simulink model "P2_SIL_Model_Diag"  (R2016a)
settings: Solver=ode2  StartTime=0.0  StopTime=Cycle_End  RelTol=1e-3
undefined symbols (not defined in the file): air, APP1_OOR, APP2_OOR, APP_Conversion_IN, APP_Mismatch, bms_inletair_temp, bms_maxchargecurrent, bms_maxdischargecurrent, BMS_Notfallkuehlung, BPP_Flt, cal, clt, ClutchEngag, CrankRequest, dcdc, eng, Engine, EngOverTemp, ENGTRQ_MSMCH_Degraded_CP, ENGTRQ_MSMCH_ErrCritical_CP, ENGTRQ_MSMCH_LimpHome_CP, EngTrqMismatch, env, ess, ESS, ESSOverTemp, fd, FFD, g, gb, Grade, IMG, KeyPos_Flt, KeyPosition, lib_APP_Conversion_IN, lib_ESS_plant_V1_2, lib_OBC_Manager, LossCAN, max_vehicle_rad_air_flow, MCUOverTemp, mot, MotDirMismatch, MotOverTemp, MotTrqMismatch, mph2kph, mph2ms, NeutralGear, obc, OBC_Manager, ParkGear, PRNDL_Flt, ReverseGear, RFD, rho, ShiftLeverPosition, sigbuilder_block, Speed, t_amb, time, tloop ... (+2)
libraries: simulink x104, EC2_libraries x12, Diagnostic x11, lib_CANerror_Detect x3, Utility x1
(part 10 of 11)

== system P2_SIL_Model_Diag/Controller/HSC/Camaro Fault Detection/Input Conversions/MCU_Conversions/Override  rollingAliveCnt [123] ==
  note: Override Switch Subsystem
  note: This subsystem is used to override the model value of a signal to a constant value
  In1 : Inport
  Multiport Switch : MultiPortSwitch  DataPortOrder=Zero-based contiguous  Inputs=2  zeroidx=on
  Override Value : Constant  Value=0  OutDataTypeStr=double
  Signal Override Switch 0 = Use Model 1 = Use Constant : Constant  Value=0
  Out1 : Outport
  wires:
  Override Value/1 -> Multiport Switch/3
  Multiport Switch/1 -> Out1/1
  In1/1 -> Multiport Switch/2
  Signal Override Switch 0 = Use Model 1 = Use Constant/1 -> Multiport Switch/1

== system P2_SIL_Model_Diag/Controller/HSC/Camaro Fault Detection/Input Conversions/TCM_Conversions/Override  rollingAliveCnt [123] ==
  note: This subsystem is used to override the model value of a signal to a constant value
  note: Override Switch Subsystem
  In1 : Inport
  Multiport Switch : MultiPortSwitch  DataPortOrder=Zero-based contiguous  Inputs=2  zeroidx=on
  Override Value : Constant  Value=0  OutDataTypeStr=double
  Signal Override Switch 0 = Use Model 1 = Use Constant : Constant  Value=0
  Out1 : Outport
  wires:
  Signal Override Switch 0 = Use Model 1 = Use Constant/1 -> Multiport Switch/1
  In1/1 -> Multiport Switch/2
  Multiport Switch/1 -> Out1/1
  Override Value/1 -> Multiport Switch/3

== system P2_SIL_Model_Diag/Controller/HSC/Camaro Fault Detection/Input Conversions/TCM_Conversions/TCM_Rolling ==
  Constant8 : Constant
  Rolling Alive Counter1 : Stateflow chart  TreatAsAtomicUnit=on
  Switch1 : Switch  Criteria=u2 > Threshold
  Out1 : Outport
  wires:
  Switch1/1 -> Out1/1  "TCMRollingAliveCnt [0 1 2 3]"
  [TCM_CAN_fault] -> Switch1/2
  Rolling Alive Counter1/1(RollingAliveCnt) -> Switch1/3
  Constant8/1 -> Switch1/1

== system P2_SIL_Model_Diag/Controller/HSC/Camaro Fault Detection/Signal Diagnostic/Clutch Signal Diagnostic/Override  Engage ==
  note: This subsystem is used to override the model value of a signal to a constant value
  note: Override Switch Subsystem
  In1 : Inport
  Multiport Switch : MultiPortSwitch  DataPortOrder=Zero-based contiguous  Inputs=2  zeroidx=on
  Override Value : Constant  Value=0  OutDataTypeStr=double
  Signal Override Switch 0 = Use Model 1 = Use Constant : Constant
  Out1 : Outport
  wires:
  Signal Override Switch 0 = Use Model 1 = Use Constant/1 -> Multiport Switch/1
  In1/1 -> Multiport Switch/2
  Multiport Switch/1 -> Out1/1
  Override Value/1 -> Multiport Switch/3

== system P2_SIL_Model_Diag/Controller/HSC/Camaro Fault Detection/Signal Diagnostic/Clutch Signal Diagnostic/Rolling Alive Counter Detection ==
  In1 : Inport
  Chart : Stateflow chart  TreatAsAtomicUnit=on
  Constant : Constant  Value=0.01
  Detect Change : simulink/Logic and Bit Operations/Detect Change  vinit=1  InputProcessing=Inherited  OutDataTypeStr=boolean
  Out1 : Outport
  wires:
  In1/1 -> Detect Change/1
  Detect Change/1 -> Chart/1(PulseDetect)
  Chart/1(flag) -> Out1/1
  Constant/1 -> Chart/2(CycleTime)

== system P2_SIL_Model_Diag/Controller/HSC/Camaro Fault Detection/Signal Diagnostic/Driver Signal Diagnostic/APP_Crosscheck ==
  In1 : Inport
  In2 : Inport  Port=2
  Abs : Abs
  Compare To Constant : simulink/Logic and Bit Operations/Compare To Constant  relop=<=  const=0.1  OutDataTypeStr=boolean
  Sum : Sum  Inputs=+-
  Out1 : Outport
  wires:
  Sum/1 -> Abs/1
  Abs/1 -> Compare To Constant/1
  In1/1 -> Sum/1
  In2/1 -> Sum/2
  Compare To Constant/1 -> Out1/1  "Drv_APP_Agree"

== system P2_SIL_Model_Diag/Controller/HSC/Camaro Fault Detection/Signal Diagnostic/Driver Signal Diagnostic/Braking fail to decelerate ==
  In1 : Inport
  In2 : Inport  Port=2
  Compare To Constant : simulink/Logic and Bit Operations/Compare To Constant  relop=~=  const=50  OutDataTypeStr=boolean
  Constant2 : Constant  Value=0
  Gain : Gain  Gain=1/13
  Gain1 : Gain  Gain=10
  Relational Operator : RelationalOperator  Operator=>  OutDataTypeStr=boolean
  Switch : Switch  Threshold=1
  Out1 : Outport
  wires:
  Relational Operator/1 -> Out1/1
  In2/1 -> Switch/1
  In1/1 -> Compare To Constant/1
  Compare To Constant/1 -> Switch/2
  [chas_plant_lin_accel] -> Gain1/1
  Gain/1 -> Relational Operator/1
  Gain1/1 -> Relational Operator/2
  Switch/1 -> Gain/1  "0-20"
  Constant2/1 -> Switch/3

== system P2_SIL_Model_Diag/Controller/HSC/Camaro Fault Detection/Signal Diagnostic/Driver Signal Diagnostic/Latch ==
  In1 : Inport
  In2 : Inport  Port=2
  Memory : Memory
  NOT : Logic  Operator=NOT  OutDataTypeStr=boolean
  OR : Logic  OutDataTypeStr=boolean
  OR1 : Logic  Operator=OR  OutDataTypeStr=boolean
  Out1 : Outport
  wires:
  In1/1 -> OR1/1
  OR/1 -> OR1/2
  OR1/1 -> Out1/1, Memory/1
  NOT/1 -> OR/1
  Memory/1 -> OR/2
  In2/1 -> NOT/1

== system P2_SIL_Model_Diag/Controller/HSC/Camaro Fault Detection/Signal Diagnostic/ESS Signal Diagnostic/Rolling Alive Counter Detection ==
  In1 : Inport
  Chart : Stateflow chart  TreatAsAtomicUnit=on
  Constant : Constant  Value=0.01
  Constant1 : Constant  Value=0.01
  Detect Change : simulink/Logic and Bit Operations/Detect Change  vinit=1  InputProcessing=Inherited  OutDataTypeStr=boolean
  Out1 : Outport
  wires:
  Constant/1 -> Chart/2(CycleTime)
  Chart/1(flag) -> Out1/1
  Detect Change/1 -> Chart/1(PulseDetect)
  In1/1 -> Detect Change/1
  Constant1/1 -> Chart/3(tloop)

== system P2_SIL_Model_Diag/Controller/HSC/Camaro Fault Detection/Signal Diagnostic/ESS Signal Diagnostic/essSOCValidity_Check ==
  In1 : Inport
  Above Normal Operation : simulink/Logic and Bit Operations/Compare To Constant  relop===  const=3  OutDataTypeStr=boolean
  Below Normal Operation : simulink/Logic and Bit Operations/Compare To Constant  relop===  const=0  OutDataTypeStr=boolean
  Logical Operator : Logic  Operator=OR  AllPortsSameDT=off  OutDataTypeStr=boolean
  Logical Operator1 : Logic  Operator=NOT  AllPortsSameDT=off  OutDataTypeStr=boolean
  Out1 : Outport
  wires:
  Logical Operator1/1 -> Out1/1
  Above Normal Operation/1 -> Logical Operator/2
  Below Normal Operation/1 -> Logical Operator/1
  Logical Operator/1 -> Logical Operator1/1
  In1/1 -> Below Normal Operation/1, Above Normal Operation/1

== system P2_SIL_Model_Diag/Controller/HSC/Camaro Fault Detection/Signal Diagnostic/ESS Signal Diagnostic/essTsignalValidity_Check ==
  In1 : Inport
  Above Normal Operation : simulink/Logic and Bit Operations/Compare To Constant  relop===  const=4  OutDataTypeStr=boolean
  Below Normal Operation : simulink/Logic and Bit Operations/Compare To Constant  relop===  const=0  OutDataTypeStr=boolean
  Logical Operator : Logic  Operator=OR  AllPortsSameDT=off  OutDataTypeStr=boolean
  Logical Operator1 : Logic  Operator=NOT  AllPortsSameDT=off  OutDataTypeStr=boolean
  Out1 : Outport
  wires:
  In1/1 -> Above Normal Operation/1, Below Normal Operation/1
  Logical Operator/1 -> Logical Operator1/1
  Below Normal Operation/1 -> Logical Operator/1
  Above Normal Operation/1 -> Logical Operator/2
  Logical Operator1/1 -> Out1/1

== system P2_SIL_Model_Diag/Controller/HSC/Camaro Fault Detection/Signal Diagnostic/Engine Signal Diagnostic/EngTempValidity_Check ==
  In1 : Inport
  Above Normal Operation : simulink/Logic and Bit Operations/Compare To Constant  relop===  const=3  OutDataTypeStr=boolean
  Logical Operator1 : Logic  Operator=NOT  AllPortsSameDT=off  OutDataTypeStr=boolean
  Out1 : Outport
  wires:
  In1/1 -> Above Normal Operation/1
  Above Normal Operation/1 -> Logical Operator1/1
  Logical Operator1/1 -> Out1/1

== system P2_SIL_Model_Diag/Controller/HSC/Camaro Fault Detection/Signal Diagnostic/Engine Signal Diagnostic/Rolling Alive Counter Detection1 ==
  In1 : Inport
  Chart : Stateflow chart  TreatAsAtomicUnit=on
  Constant : Constant  Value=0.01
  Detect Change : simulink/Logic and Bit Operations/Detect Change  vinit=1  InputProcessing=Inherited  OutDataTypeStr=boolean
  Out1 : Outport
  wires:
  In1/1 -> Detect Change/1
  Detect Change/1 -> Chart/1(PulseDetect)
  Chart/1(flag) -> Out1/1
  Constant/1 -> Chart/2(CycleTime)

== system P2_SIL_Model_Diag/Controller/HSC/Camaro Fault Detection/Signal Diagnostic/Motor Signal Diagnostic/Rolling Alive Counter Detection ==
  In1 : Inport
  Chart : Stateflow chart  TreatAsAtomicUnit=on
  Constant : Constant  Value=0.01
  Detect Change : simulink/Logic and Bit Operations/Detect Change  vinit=1  InputProcessing=Inherited  OutDataTypeStr=boolean
  Out1 : Outport
  wires:
  Constant/1 -> Chart/2(CycleTime)
  Chart/1(flag) -> Out1/1
  Detect Change/1 -> Chart/1(PulseDetect)
  In1/1 -> Detect Change/1

== system P2_SIL_Model_Diag/Controller/HSC/Camaro Fault Detection/Signal Diagnostic/Motor Signal Diagnostic/Subsystem ==
  ClearFault : Inport
  In2 : Inport  Port=2
  MCUTempValidityCheck : simulink/Logic and Bit Operations/Interval Test  IntervalClosedRight=on  uplimit=100  IntervalClosedLeft=on  lowlimit=-40  OutDataTypeStr=boolean
  MCUTsignalRange : Stateflow chart  TreatAsAtomicUnit=on
  MCUTemp_degC_SigValid : Outport
  MCUTempRange : Outport  Port=2
  wires:
  In2/1 -> MCUTempValidityCheck/1, MCUTsignalRange/2(signalValue)
  ClearFault/1 -> MCUTsignalRange/1(clearFaults)
  MCUTempValidityCheck/1 -> MCUTemp_degC_SigValid/1  "MCUTemp_degC_SigValid"
  MCUTsignalRange/1(MCUTempRange) -> MCUTempRange/1  "MCUTempRange[0_4]"

== system P2_SIL_Model_Diag/Controller/HSC/Camaro Fault Detection/Signal Diagnostic/Motor Signal Diagnostic/Subsystem1 ==
  ClearFault : Inport
  In2 : Inport  Port=2
  MotorTempValidityCheck : simulink/Logic and Bit Operations/Interval Test  IntervalClosedRight=on  uplimit=150  IntervalClosedLeft=on  lowlimit=-20  OutDataTypeStr=boolean
  MotorTsignalRange : Stateflow chart  TreatAsAtomicUnit=on
  MotorTemp_degC_SigValid : Outport
  MotorTempRange : Outport  Port=2
  wires:
  ClearFault/1 -> MotorTsignalRange/1(clearFaults)
  MotorTsignalRange/1(MotorTempRange) -> MotorTempRange/1  "MotorTempRange[0_4]"
  In2/1 -> MotorTempValidityCheck/1, MotorTsignalRange/2(signalValue)
  MotorTempValidityCheck/1 -> MotorTemp_degC_SigValid/1  "MotorTemp_degC_SigValid"

== system P2_SIL_Model_Diag/Controller/HSC/Camaro Fault Detection/Signal Diagnostic/Transmission Signal Diagnostic/Rolling Alive Counter Detection ==
  In1 : Inport
  Chart : Stateflow chart  TreatAsAtomicUnit=on
  Constant : Constant  Value=0.01
  Detect Change : simulink/Logic and Bit Operations/Detect Change  vinit=1  InputProcessing=Inherited  OutDataTypeStr=boolean
  Out1 : Outport
  wires:
  In1/1 -> Detect Change/1
  Detect Change/1 -> Chart/1(PulseDetect)
  Chart/1(flag) -> Out1/1
  Constant/1 -> Chart/2(CycleTime)

== system P2_SIL_Model_Diag/Controller/HSC/Camaro Fault Detection/Signal Generator /BMS_Signals/BMS_rollingAliveCnt ==
  Constant : Constant
  Rolling Alive Counter : Stateflow chart  TreatAsAtomicUnit=on
  Switch : Switch  Criteria=u2 > Threshold
  Out1 : Outport
  wires:
  Switch/1 -> Out1/1  "BMS_rollingAliveCnt [0 1 2 3]"
  [BMS_CAN_fault] -> Switch/2
  Constant/1 -> Switch/1
  Rolling Alive Counter/1(RollingAliveCnt) -> Switch/3

== system P2_SIL_Model_Diag/Controller/HSC/Camaro Fault Detection/Signal Generator /Clutch_Signals/Clutch_Rolling ==
  Constant8 : Constant
  Rolling Alive Counter1 : Stateflow chart  TreatAsAtomicUnit=on
  Switch1 : Switch  Criteria=u2 > Threshold
  Out1 : Outport
  wires:
  [Clutch_CAN_fault] -> Switch1/2
  Rolling Alive Counter1/1(RollingAliveCnt) -> Switch1/3
  Constant8/1 -> Switch1/1
  Switch1/1 -> Out1/1  "ClutchRollingAliveCnt [0 1 2 3]"

== system P2_SIL_Model_Diag/Controller/HSC/Camaro Fault Detection/Signal Generator /ECM_Signals/ECM_CAN_Rolling ==
  Constant8 : Constant
  Rolling Alive Counter1 : Stateflow chart  TreatAsAtomicUnit=on
  Switch1 : Switch  Criteria=u2 > Threshold
  Out1 : Outport
  wires:
  [ECM_CAN_fault] -> Switch1/2
  Constant8/1 -> Switch1/1
  Switch1/1 -> Out1/1  "ECMRollingAliveCnt [0 1 2 3]"
  Rolling Alive Counter1/1(RollingAliveCnt) -> Switch1/3

== system P2_SIL_Model_Diag/Controller/HSC/Camaro Fault Detection/Signal Generator /MCU_Signals/MCU_CAN_rolling ==
  Constant8 : Constant
  Rolling Alive Counter1 : Stateflow chart  TreatAsAtomicUnit=on
  Switch1 : Switch  Criteria=u2 > Threshold
  Out1 : Outport
  wires:
  Switch1/1 -> Out1/1  "MCURollingAliveCnt [0 1 2 3]"
  [MCU_CAN_fault] -> Switch1/2
  Constant8/1 -> Switch1/1
  Rolling Alive Counter1/1(RollingAliveCnt) -> Switch1/3

== system P2_SIL_Model_Diag/Controller/HSC/Camaro Fault Detection/Signal Generator /TCM_Signals/TCM_Rolling ==
  Constant8 : Constant
  Rolling Alive Counter1 : Stateflow chart  TreatAsAtomicUnit=on
  Switch1 : Switch  Criteria=u2 > Threshold
  Out1 : Outport
  wires:
  Switch1/1 -> Out1/1  "TCMRollingAliveCnt [0 1 2 3]"
  [TCM_CAN_fault] -> Switch1/2
  Rolling Alive Counter1/1(RollingAliveCnt) -> Switch1/3
  Constant8/1 -> Switch1/1

== system P2_SIL_Model_Diag/Controller/HSC/Camaro Fault Detection/SystemDiag/Combined_SystemDiagnostics/Override Combined_System Status ==
  note: Override Switch Subsystem
  note: This subsystem is used to override the model value of a signal to a constant value
  In1 : Inport
  Multiport Switch : MultiPortSwitch  DataPortOrder=Zero-based contiguous  Inputs=2  zeroidx=on
  Override Value : Constant  Value=0  OutDataTypeStr=double
  Signal Override Switch 0 = Use Model 1 = Use Constant : Constant  Value=0
  Out1 : Outport
  wires:
  Override Value/1 -> Multiport Switch/3
  Multiport Switch/1 -> Out1/1
  In1/1 -> Multiport Switch/2
  Signal Override Switch 0 = Use Model 1 = Use Constant/1 -> Multiport Switch/1

== system P2_SIL_Model_Diag/Controller/HSC/Camaro Fault Detection/SystemDiag/eSystemDiagnostics/Override eSystem Status ==
  note: This subsystem is used to override the model value of a signal to a constant value
  note: Override Switch Subsystem
  In1 : Inport
  Multiport Switch : MultiPortSwitch  DataPortOrder=Zero-based contiguous  Inputs=2  zeroidx=on
  Override Value : Constant  Value=0  OutDataTypeStr=double
  Signal Override Switch 0 = Use Model 1 = Use Constant : Constant  Value=0
  Out1 : Outport
  wires:
  Signal Override Switch 0 = Use Model 1 = Use Constant/1 -> Multiport Switch/1
  In1/1 -> Multiport Switch/2
  Multiport Switch/1 -> Out1/1
  Override Value/1 -> Multiport Switch/3

== system P2_SIL_Model_Diag/Controller/HSC/Camaro Fault Detection/SystemDiag/iceSystemDiagnostics/Override iceSystem Status ==
  note: This subsystem is used to override the model value of a signal to a constant value
  note: Override Switch Subsystem
  In1 : Inport
  Multiport Switch : MultiPortSwitch  DataPortOrder=Zero-based contiguous  Inputs=2  zeroidx=on
  Override Value : Constant  Value=2  OutDataTypeStr=double
  Signal Override Switch 0 = Use Model 1 = Use Constant : Constant  Value=0
  Out1 : Outport
  wires:
  Signal Override Switch 0 = Use Model 1 = Use Constant/1 -> Multiport Switch/1
  In1/1 -> Multiport Switch/2
  Multiport Switch/1 -> Out1/1
  Override Value/1 -> Multiport Switch/3

== system P2_SIL_Model_Diag/Controller/HSC/Driver_Requests/APP_BPP to DrvIntndAxlTrq1/Post Driver Intnded Axle Torque/Ratio Filter ==
  Ratio : Inport
  Abs : Abs
  Compare To Zero : simulink/Logic and Bit Operations/Compare To Zero  relop===  OutDataTypeStr=boolean
  Constant : Constant  Value=cal.Time.TrnsOvrllEstTrqRatioSwitch
  Mature_Delay : EC2_libraries/Mature_Delay
  Memory1 : Memory  X0=1
  Switch1 : Switch  Threshold=1
  Switch2 : Switch  Threshold=1
  Filtered_Ratio : Outport
  wires:
  Switch2/1 -> Memory1/1, Filtered_Ratio/1  "gear_ratio"
  Memory1/1 -> Switch1/3
  Mature_Delay/1 -> Switch1/2
  Constant/1 -> Mature_Delay/2
  Switch1/1 -> Switch2/1
  Abs/1 -> Switch2/3, Switch1/1
  Compare To Zero/1 -> Switch2/2, Mature_Delay/1
  Ratio/1 -> Abs/1, Compare To Zero/1

== system P2_SIL_Model_Diag/Controller/HSC/Driver_Requests/APP_BPP to DrvIntndAxlTrq2/Post Driver Intnded Axle Torque/Ratio Filter ==
  Ratio : Inport
  Abs : Abs
  Compare To Zero : simulink/Logic and Bit Operations/Compare To Zero  relop===  OutDataTypeStr=boolean
  Constant : Constant  Value=cal.Time.TrnsOvrllEstTrqRatioSwitch
  Mature_Delay : EC2_libraries/Mature_Delay
  Memory1 : Memory  X0=1
  Switch1 : Switch  Threshold=1
  Switch2 : Switch  Threshold=1
  Filtered_Ratio : Outport
  wires:
  Ratio/1 -> Compare To Zero/1, Abs/1
  Compare To Zero/1 -> Mature_Delay/1, Switch2/2
  Abs/1 -> Switch1/1, Switch2/3
  Switch1/1 -> Switch2/1
  Constant/1 -> Mature_Delay/2
  Mature_Delay/1 -> Switch1/2
  Memory1/1 -> Switch1/3
  Switch2/1 -> Filtered_Ratio/1, Memory1/1  "gear_ratio"

== system P2_SIL_Model_Diag/Controller/HSC/Powertrain Manager/HV Manager/BMS_Manager/Isolation Fault Calculation ==
  note: This block  will allows to know which HV main
      | is having issues. HV POS 25, HV NEG 23.
  Sensors : Inport
  Add : Sum
  Bus Selector5 : BusSelector  OutputSignals=from_CAN.fromEBCAN.from_BMSAntrieb.ISO_Hybrid_01_Resp_Data.ISO_Hybrid_01_Resp_Data_byte_3,from_CAN.fromEBCAN.from_BMSAntrieb.ISO_Hybrid_01_Resp_Data.ISO_Hybrid_01_Resp_Data_byte_4,from_CAN.fromEBCAN.from_BMSAntrieb.ISO_Hybrid_01_Resp_Data.ISO_Hybrid_01_Resp_Data_byte_5
  HVnegativeISO : Constant  Value=0
  HVpositiveISO : Constant
  ISOfault : Constant
  ISOmultiplier : Constant  Value=256
  ISOnofault : Constant  Value=0
  Minimum Allowed Isolation Resistance : Switch  Criteria=u2 > Threshold  Threshold=500000
  POS or NEG HV MAIN : Switch  Criteria=u2 > Threshold  Threshold=24
  Product : Product
  Product1 : Product
  Resistance Adjustment : Constant  Value=1000
  Terminator8 : Terminator
  tag scope: IsolationFault=global
  wires:
  Bus Selector5/1 -> POS or NEG HV MAIN/2  "<ISO_Hybrid_01_Resp_Data_byte_3>"
  HVpositiveISO/1 -> POS or NEG HV MAIN/1
  HVnegativeISO/1 -> POS or NEG HV MAIN/3
  POS or NEG HV MAIN/1 -> Terminator8/1
  ISOmultiplier/1 -> Product/2
  Bus Selector5/2 -> Product/1  "<ISO_Hybrid_01_Resp_Data_byte_4>"
  Bus Selector5/3 -> Add/2  "<ISO_Hybrid_01_Resp_Data_byte_5>"
  Product/1 -> Add/1
  Add/1 -> Product1/1
  ISOnofault/1 -> Minimum Allowed Isolation Resistance/1
  ISOfault/1 -> Minimum Allowed Isolation Resistance/3
  Product1/1 -> Minimum Allowed Isolation Resistance/2
  Resistance Adjustment/1 -> Product1/2
  Minimum Allowed Isolation Resistance/1 -> [IsolationFault]
  Sensors/1 -> Bus Selector5/1

== system P2_SIL_Model_Diag/Controller/HSC/Powertrain Manager/Torque Distribution/AxlTrq_to_EngTrq1/Ratio Filter ==
  Ratio : Inport
  Abs : Abs
  Compare To Zero : simulink/Logic and Bit Operations/Compare To Zero  relop===  OutDataTypeStr=boolean
  Constant : Constant  Value=cal.Time.TrnsOvrllEstTrqRatioSwitch
  Mature_Delay : EC2_libraries/Mature_Delay
  Memory1 : Memory  X0=1
  Switch1 : Switch  Threshold=1
  Switch2 : Switch  Threshold=1
  Filtered_Ratio : Outport
  wires:
  Switch2/1 -> Memory1/1, Filtered_Ratio/1  "gear_ratio"
  Memory1/1 -> Switch1/3
  Mature_Delay/1 -> Switch1/2
  Constant/1 -> Mature_Delay/2
  Switch1/1 -> Switch2/1
  Abs/1 -> Switch2/3, Switch1/1
  Compare To Zero/1 -> Switch2/2, Mature_Delay/1
  Ratio/1 -> Abs/1, Compare To Zero/1

== system P2_SIL_Model_Diag/Controller/HSC/Powertrain Manager/Torque Distribution/AxlTrq_to_EngTrq2/Ratio Filter ==
  Ratio : Inport
  Abs : Abs
  Compare To Zero : simulink/Logic and Bit Operations/Compare To Zero  relop===  OutDataTypeStr=boolean
  Constant : Constant  Value=cal.Time.TrnsOvrllEstTrqRatioSwitch
  Mature_Delay : EC2_libraries/Mature_Delay
  Memory1 : Memory  X0=1
  Switch1 : Switch  Threshold=1
  Switch2 : Switch  Threshold=1
  Filtered_Ratio : Outport
  wires:
  Ratio/1 -> Compare To Zero/1, Abs/1
  Compare To Zero/1 -> Mature_Delay/1, Switch2/2
  Abs/1 -> Switch1/1, Switch2/3
  Switch1/1 -> Switch2/1
  Constant/1 -> Mature_Delay/2
  Mature_Delay/1 -> Switch1/2
  Memory1/1 -> Switch1/3
  Switch2/1 -> Filtered_Ratio/1, Memory1/1  "gear_ratio"

== system P2_SIL_Model_Diag/Controller/HSC/Powertrain Manager/Torque Distribution/AxlTrq_to_MtrTrq1/Ratio Filter ==
  Ratio : Inport
  Abs : Abs
  Compare To Zero : simulink/Logic and Bit Operations/Compare To Zero  relop===  OutDataTypeStr=boolean
  Constant : Constant  Value=cal.Time.TrnsOvrllEstTrqRatioSwitch
  Mature_Delay : EC2_libraries/Mature_Delay
  Memory1 : Memory  X0=1
  Switch1 : Switch  Threshold=1
  Switch2 : Switch  Threshold=1
  Filtered_Ratio : Outport
  wires:
  Switch2/1 -> Memory1/1, Filtered_Ratio/1  "gear_ratio"
  Memory1/1 -> Switch1/3
  Mature_Delay/1 -> Switch1/2
  Constant/1 -> Mature_Delay/2
  Switch1/1 -> Switch2/1
  Abs/1 -> Switch2/3, Switch1/1
  Compare To Zero/1 -> Switch2/2, Mature_Delay/1
  Ratio/1 -> Abs/1, Compare To Zero/1

== system P2_SIL_Model_Diag/Controller/HSC/Powertrain Manager/Torque Distribution/AxlTrq_to_MtrTrq2/Ratio Filter ==
  Ratio : Inport
  Abs : Abs
  Compare To Zero : simulink/Logic and Bit Operations/Compare To Zero  relop===  OutDataTypeStr=boolean
  Constant : Constant  Value=cal.Time.TrnsOvrllEstTrqRatioSwitch
  Mature_Delay : EC2_libraries/Mature_Delay
  Memory1 : Memory  X0=1
  Switch1 : Switch  Threshold=1
  Switch2 : Switch  Threshold=1
  Filtered_Ratio : Outport
  wires:
  Ratio/1 -> Compare To Zero/1, Abs/1
  Compare To Zero/1 -> Mature_Delay/1, Switch2/2
  Abs/1 -> Switch1/1, Switch2/3
  Switch1/1 -> Switch2/1
  Constant/1 -> Mature_Delay/2
  Mature_Delay/1 -> Switch1/2
  Memory1/1 -> Switch1/3
  Switch2/1 -> Filtered_Ratio/1, Memory1/1  "gear_ratio"

== system P2_SIL_Model_Diag/Controller/HSC/Powertrain Manager/Torque Distribution/Supervisory  Control  Logic1/VehReady.CD_Limited.MotTrqCalc1/Motor Troque Mismatch Mitigation ==
  In1 : Inport
  MotTrqMismchDegraded : Inport  Port=2
  MotTrqMismchLimp : Inport  Port=3
  Constant5 : Constant  Value=mot.plant.init.trq_posmax
  Gain1 : Gain  Gain=cal.DegradedPerc
  Gain3 : Gain  Gain=cal.LimpHPerc
  Min1 : MinMax  Inputs=2
  Min2 : MinMax  Inputs=2
  Switch1 : Switch  Threshold=1
  Switch2 : Switch  Threshold=1
  Unit Delay : UnitDelay  SampleTime=-1
  Unit Delay1 : UnitDelay  SampleTime=-1
  Out1 : Outport
  wires:
  MotTrqMismchDegraded/1 -> Unit Delay/1
  Switch2/1 -> Out1/1
  MotTrqMismchLimp/1 -> Unit Delay1/1
  In1/1 -> Switch1/3, Min2/1, Min1/2
  Min1/1 -> Switch2/1  "LimpHome_MotTrq"
  Gain3/1 -> Min1/1
  Gain1/1 -> Min2/2
  Min2/1 -> Switch1/1  "Degraded_MotTrq"
  Unit Delay/1 -> Switch1/2
  Unit Delay1/1 -> Switch2/2
  Switch1/1 -> Switch2/3
  Constant5/1 -> Gain1/1, Gain3/1

== system P2_SIL_Model_Diag/Controller/HSC/Powertrain Manager/Torque Distribution/Supervisory  Control  Logic1/VehReady.CD_Limited.MotTrqCalc1/OverTemperature Mitigation ==
  In1 : Inport
  essTempRange : Inport  Port=2
  MCUTempRange : Inport  Port=3
  MotorTempRange : Inport  Port=4
  Compare To Constant : simulink/Logic and Bit Operations/Compare To Constant  relop===  const=1  OutDataTypeStr=boolean
  Compare To Constant1 : simulink/Logic and Bit Operations/Compare To Constant  relop===  const=3  OutDataTypeStr=boolean
  Compare To Constant2 : simulink/Logic and Bit Operations/Compare To Constant  relop===  const=1  OutDataTypeStr=boolean
  Compare To Constant3 : simulink/Logic and Bit Operations/Compare To Constant  relop===  const=3  OutDataTypeStr=boolean
  Compare To Constant4 : simulink/Logic and Bit Operations/Compare To Constant  relop===  const=1  OutDataTypeStr=boolean
  Compare To Constant5 : simulink/Logic and Bit Operations/Compare To Constant  relop===  const=3  OutDataTypeStr=boolean
  Constant3 : Constant  Value=mot.plant.init.trq_posmax
  Constant5 : Constant  Value=mot.plant.init.trq_posmax
  Gain1 : Gain  Gain=0.4
  Gain3 : Gain  Gain=0.5
  Logical Operator : Logic  Operator=OR  AllPortsSameDT=off  OutDataTypeStr=boolean
  Logical Operator1 : Logic  Operator=OR  AllPortsSameDT=off  OutDataTypeStr=boolean
  Logical Operator2 : Logic  Operator=OR  AllPortsSameDT=off  OutDataTypeStr=boolean
  MinMax1 : MinMax  Inputs=2
  MinMax2 : MinMax  Inputs=2
  Switch1 : Switch  Threshold=1
  Switch2 : Switch  Threshold=1
  Switch3 : Switch  Threshold=1
  Out1 : Outport
  wires:
  MotorTempRange/1 -> Compare To Constant5/1, Compare To Constant4/1
  Constant5/1 -> Gain3/1
  Logical Operator1/1 -> Switch2/2
  Compare To Constant1/1 -> Logical Operator/2
  Compare To Constant/1 -> Logical Operator/1
  Constant3/1 -> Gain1/1
  MinMax2/1 -> Switch3/1, Switch2/1
  MinMax1/1 -> Switch1/1
  Logical Operator/1 -> Switch1/2
  Logical Operator2/1 -> Switch3/2
  In1/1 -> MinMax2/1, Switch1/3, MinMax1/1
  Gain1/1 -> MinMax2/2
  Gain3/1 -> MinMax1/2
  Switch2/1 -> Switch3/3
  MCUTempRange/1 -> Compare To Constant3/1, Compare To Constant2/1
  Compare To Constant2/1 -> Logical Operator1/1
  Compare To Constant3/1 -> Logical Operator1/2
  essTempRange/1 -> Compare To Constant1/1, Compare To Constant/1
  Switch1/1 -> Switch2/3
  Compare To Constant4/1 -> Logical Operator2/1
  Compare To Constant5/1 -> Logical Operator2/2
  Switch3/1 -> Out1/1

== system P2_SIL_Model_Diag/Controller/HSC/Powertrain Manager/Torque Distribution/Supervisory  Control  Logic1/VehReady.Eng_Only_Mode.EngTrqCalc/Subsystem ==
  In1 : Inport
  EngTrqMismchDegraded : Inport  Port=2
  EngTrqMismchLimp : Inport  Port=3
  Eng_TempRange : Inport  Port=4
  iceSystemStatus : Inport  Port=5
  Compare To Constant : simulink/Logic and Bit Operations/Compare To Constant  relop===  const=1  OutDataTypeStr=boolean
  Eng Troque Mismatch Mitigation : Subsystem
  OverTemperature Mitigation : Subsystem
  Switch2 : Switch  Threshold=1
  Out1 : Outport
  wires:
  Switch2/1 -> Out1/1
  Compare To Constant/1 -> Switch2/2
  EngTrqMismchLimp/1 -> Eng Troque Mismatch Mitigation/3(EngTrqMismchLimp)
  EngTrqMismchDegraded/1 -> Eng Troque Mismatch Mitigation/2(EngTrqMismchDegraded)
  Eng_TempRange/1 -> OverTemperature Mitigation/2(essTempRange)
  Eng Troque Mismatch Mitigation/1(Out1) -> OverTemperature Mitigation/1(In1)
  In1/1 -> Eng Troque Mismatch Mitigation/1(In1), Switch2/3
  iceSystemStatus/1 -> Compare To Constant/1
  OverTemperature Mitigation/1(Out1) -> Switch2/1

== system P2_SIL_Model_Diag/Camaro Plant Model/ESS/Soft BMS/Limits/Average Current/60 sec rolling average1/1sec trigger ==
  0 : Constant  Value=0
  Compare To Constant : simulink/Logic and Bit Operations/Compare To Constant  relop=<=  const=3.0  OutDataTypeStr=boolean
  Data Type Conversion : DataTypeConversion
  Sum2 : Sum  Inputs=|++
  Switch : Switch  Threshold=0.5
  accumulate2 : Memory  InheritSampleTime=on
  tloop : Constant  Value=tloop
  Trigger : Outport
  wires:
  Data Type Conversion/1 -> Trigger/1, Switch/2
  0/1 -> Switch/1
  Compare To Constant/1 -> Data Type Conversion/1
  Switch/1 -> accumulate2/1
  Sum2/1 -> Switch/3, Compare To Constant/1
  accumulate2/1 -> Sum2/2
  tloop/1 -> Sum2/1

== system P2_SIL_Model_Diag/Camaro Plant Model/ESS/Soft BMS/Limits/Average Current/60 sec rolling average1/60 sec average ==
  1sec : Inport
  Enable : EnablePort
  60 second : Delay  DelayLength=60  InputProcessing=Inherited  SampleTime=tloop
  Gain2 : Gain  Gain=1/60
  Sum2 : Sum  Inputs=++-
  accumulate2 : Memory  InheritSampleTime=on
  Average : Outport
  wires:
  1sec/1 -> Sum2/2, 60 second/1
  Gain2/1 -> Average/1
  accumulate2/1 -> Sum2/1
  60 second/1 -> Sum2/3
  Sum2/1 -> Gain2/1, accumulate2/1

== system P2_SIL_Model_Diag/Camaro Plant Model/ESS/Soft BMS/Limits/Average Current/60 sec rolling average2/1sec trigger ==
  0 : Constant  Value=0
  Compare To Constant : simulink/Logic and Bit Operations/Compare To Constant  relop=<=  const=3.0  OutDataTypeStr=boolean
  Data Type Conversion : DataTypeConversion
  Sum2 : Sum  Inputs=|++
  Switch : Switch  Threshold=0.5
  accumulate2 : Memory  InheritSampleTime=on
  tloop : Constant  Value=tloop
  Trigger : Outport
  wires:
  Data Type Conversion/1 -> Trigger/1, Switch/2
  0/1 -> Switch/1
  Compare To Constant/1 -> Data Type Conversion/1
  Switch/1 -> accumulate2/1
  Sum2/1 -> Switch/3, Compare To Constant/1
  accumulate2/1 -> Sum2/2
  tloop/1 -> Sum2/1

== system P2_SIL_Model_Diag/Camaro Plant Model/ESS/Soft BMS/Limits/Average Current/60 sec rolling average2/60 sec average ==
  1sec : Inport
  Enable : EnablePort
  60 second : Delay  DelayLength=60  InputProcessing=Inherited  SampleTime=tloop
  Gain2 : Gain  Gain=1/60
  Sum2 : Sum  Inputs=++-
  accumulate2 : Memory  InheritSampleTime=on
  Average : Outport
  wires:
  1sec/1 -> Sum2/2, 60 second/1
  Gain2/1 -> Average/1
  accumulate2/1 -> Sum2/1
  60 second/1 -> Sum2/3
  Sum2/1 -> Gain2/1, accumulate2/1

== system P2_SIL_Model_Diag/Camaro Plant Model/IMG/Soft MCU/Torque Calculation/max torque /Heat index/Divide ==
  note: Take care of
      | division by 0
  numerator : Inport
  denominator : Inport  Port=2
  Fcn : Fcn  Expr=u[1] / ( u[2] + eps*(u[2]==0) )
  Mux : Mux  Inputs=2
  quotient : Outport
  wires:
  denominator/1 -> Mux/2
  Fcn/1 -> quotient/1
  numerator/1 -> Mux/1
  Mux/1 -> Fcn/1

== system P2_SIL_Model_Diag/Camaro Plant Model/Transmission1/Transmission Plant/Gearbox/Speed Calculation/P//N/Subsystem2 ==
  In1 : Inport
  In2 : Inport  Port=2
  Fcn : Fcn  Expr=u[1]/(u[2]+eps)*(u[2]!=0)
  Mux : Mux  Inputs=2
  Out1 : Outport
  wires:
  Mux/1 -> Fcn/1
  In1/1 -> Mux/1
  Fcn/1 -> Out1/1
  In2/1 -> Mux/2

== system P2_SIL_Model_Diag/Camaro Plant Model/Transmission1/Transmission Plant/Gearbox/Speed Calculation/P//N/input shaft free wheeling losses ==
  input shaft speed : Inport
  Constant1 : Constant  Value=0
  Fcn1 : Fcn  Expr=u==0
  Gain1 : Gain  Gain=0.08  SaturateOnIntegerOverflow=on  OutDataTypeStr=Inherit: Same as input  ParamDataTypeStr=Inherit: Same as input
  Switch2 : Switch  Threshold=0.5  SaturateOnIntegerOverflow=on  InputSameDT=on
  input shaft decel : Outport
  wires:
  input shaft speed/1 -> Switch2/3, Fcn1/1
  Fcn1/1 -> Switch2/2
  Gain1/1 -> input shaft decel/1
  Switch2/1 -> Gain1/1
  Constant1/1 -> Switch2/1

== system P2_SIL_Model_Diag/Camaro Plant Model/Transmission1/Transmission Plant/Gearbox/Speed Calculation/R//D/S-R Flip-Flop ==
  S : Inport
  R : Inport  Port=2
  Demux : Demux  Outputs=2
  Logic : CombinatorialLogic  TruthTable=[0 1;0 1;1 0;0 1;1 0;0 1;1 0;1 0]
  Memory : Memory  X0=initial_condition  InheritSampleTime=on
  Mux : Mux  Inputs=3
  Q : Outport  InitialOutput=0
  !Q : Outport  Port=2  InitialOutput=1
  wires:
  R/1 -> Mux/3
  S/1 -> Mux/2
  Memory/1 -> Mux/1
  Demux/1 -> Memory/1, Q/1
  Demux/2 -> !Q/1
  Logic/1 -> Demux/1
  Mux/1 -> Logic/1

== system P2_SIL_Model_Diag/Camaro Plant Model/Transmission1/Transmission Plant/Torque Converter/Torque Calculation/spd and trq ratio/speed ratio ==
  note: Take care of
      | division by 0
  numerator : Inport
  denominator : Inport  Port=2
  Fcn : Fcn  Expr=u[1] / ( u[2] + eps*(u[2]==0) )
  Mux : Mux  Inputs=2
  quotient : Outport
  wires:
  denominator/1 -> Mux/2
  Fcn/1 -> quotient/1
  numerator/1 -> Mux/1
  Mux/1 -> Fcn/1

== system P2_SIL_Model_Diag/Controller/HSC/Camaro Fault Detection/Component Diagnostic/Motor Component Diagnostic/Torque_Mismatch/Latch ==
  In1 : Inport
  In2 : Inport  Port=2
  Memory : Memory
  NOT : Logic  Operator=NOT  OutDataTypeStr=boolean
  OR : Logic  OutDataTypeStr=boolean
  OR1 : Logic  Operator=OR  OutDataTypeStr=boolean
  Out1 : Outport
  wires:
  In1/1 -> OR1/1
  OR/1 -> OR1/2
  OR1/1 -> Out1/1, Memory/1
  NOT/1 -> OR/1
  Memory/1 -> OR/2
  In2/1 -> NOT/1

== system P2_SIL_Model_Diag/Controller/HSC/Powertrain Manager/Torque Distribution/Supervisory  Control  Logic1/VehReady.Eng_Only_Mode.EngTrqCalc/Subsystem/Eng Troque Mismatch Mitigation ==
  In1 : Inport
  EngTrqMismchDegraded : Inport  Port=2
  EngTrqMismchLimp : Inport  Port=3
  Constant5 : Constant  Value=eng.plant.eng_max_torque
  Gain1 : Gain  Gain=cal.DegradedPerc
  Gain3 : Gain  Gain=cal.LimpHPerc
  Min1 : MinMax  Inputs=2
  Min2 : MinMax  Inputs=2
  Switch1 : Switch  Threshold=1
  Switch2 : Switch  Threshold=1
  Unit Delay : UnitDelay  SampleTime=-1
  Unit Delay1 : UnitDelay  SampleTime=-1
  Out1 : Outport
  wires:
  EngTrqMismchDegraded/1 -> Unit Delay/1
  Switch2/1 -> Out1/1
  EngTrqMismchLimp/1 -> Unit Delay1/1
  In1/1 -> Switch1/3, Min2/1, Min1/2
  Min1/1 -> Switch2/1  "LimpHome_EngTrq"
  Gain3/1 -> Min1/1
  Gain1/1 -> Min2/2
  Min2/1 -> Switch1/1  "Degraded_EngTrq"
  Unit Delay/1 -> Switch1/2
  Unit Delay1/1 -> Switch2/2
  Switch1/1 -> Switch2/3
  Constant5/1 -> Gain1/1, Gain3/1

== system P2_SIL_Model_Diag/Controller/HSC/Powertrain Manager/Torque Distribution/Supervisory  Control  Logic1/VehReady.Eng_Only_Mode.EngTrqCalc/Subsystem/OverTemperature Mitigation ==
  In1 : Inport
  essTempRange : Inport  Port=2
  Compare To Constant : simulink/Logic and Bit Operations/Compare To Constant  relop===  const=2  OutDataTypeStr=boolean
  Constant5 : Constant  Value=mot.plant.init.trq_posmax
  Gain3 : Gain  Gain=0.5
  MinMax1 : MinMax  Inputs=2
  Switch1 : Switch  Threshold=1
  Out1 : Outport
  wires:
  Constant5/1 -> Gain3/1
  MinMax1/1 -> Switch1/1
  Compare To Constant/1 -> Switch1/2
  In1/1 -> Switch1/3, MinMax1/1
  Gain3/1 -> MinMax1/2
  essTempRange/1 -> Compare To Constant/1
  Switch1/1 -> Out1/1

== stateflow chart P2_SIL_Model_Diag/Camaro Plant Model/ESS/Soft BMS/State Machine/Startup_Shutdown_EPO_Sequence ==
  state BCM_ON
    state Default_Error_State
      en: BMS_Init_abgeschlossen=0;
      BMS_IstModus=5;
    state Standby
      en: BMS_Init_abgeschlossen=0;
      BMS_IstModus=0;
    state Normal_Driving
      en: NHM_BMS_Car_WakeUp=1;
      BMS_IstModus=1;
      BMS_Init_abgeschlossen=1;
      during: timer++;
    state Charging
      en:BMS_IstModus=4;
      BMS_Init_abgeschlossen =1;
      during: timer++;
    (default) -> Default_Error_State : [T_15&&T_30]
    Default_Error_State -> Standby : [Diag_Rq_Fktnl_Data_OBD==1]
        | %ErrorClear
    Standby -> Charging [order 1] : [MO_BMS_Sollmodus==4]
        | %Standby>Charging
    Standby -> Normal_Driving [order 2] : [MO_BMS_Sollmodus==1]
        | {timer=0;}
        | %Standby>NormalDriving
    Normal_Driving -> Standby [order 1] : [MO_BMS_Sollmodus==0]
        | %NormalDriving>Standby
    Charging -> Standby [order 1] : [MO_BMS_Sollmodus==0]
        | %Charging>Standby
    Normal_Driving -> Charging [order 2] : [MO_BMS_Sollmodus==4] %NormalDriving>Charging
    Charging -> Normal_Driving [order 2] : [MO_BMS_Sollmodus==1] %Charging>NormalDriving
  state BCM_OFF
    state Prepare_to_Sleep
      en: NMH_BMS_Start_2=0;
      BMS_IstModus=5;
    state Ready_to_Sleep
      en: NMH_BMS_Normal_Mode_2=0;
      BMS_SleepInd=1;
      BMS_IstModus=5;
    state Bus_Sleep
      en: NMH_BMS_Start_1=0;
      BMS_SleepInd=1;
      BMS_IstModus=5;
    (default) -> Prepare_to_Sleep
    Prepare_to_Sleep -> Ready_to_Sleep : [timer>=0.05/tloop]
    Ready_to_Sleep -> Bus_Sleep : [timer>=0.05/tloop]
  note: !(veh_wake||chga_wake) || ...
      | !hsc_bcm_enable && !bcm_mainc_stat && bcm_cpwr_cmd]
  state EPO1
    BMS_Fehler_HS_offen=1;
    BMS_Fehler_HS_verschweisst =1;
    BMS_Fehler_HVBatt_Abschaltung=1;
    BMS_Fehler_HVBatt_Abschaltung_Anf=1;
    BMS_IstModus=5;
  state EPO
    BMS_Fehler_Notabschaltung_Crash=1;
    BMS_Fehler_Notabschaltung_Pilot=1;
    BMS_Fehler_Pilot=1;
    BMS_IstModus=5;
  (default) -> BCM_OFF
  BCM_OFF -> BCM_ON : [T_15&&T_30]
  BCM_ON -> BCM_OFF [order 1] : [T_15==0&&T_30==0]
  BCM_ON -> EPO1 [order 2] : [BattError]
  EPO1 -> BCM_OFF : [T_15==0&&T_30==0]
  EPO -> BCM_OFF : [T_15==0&&T_30==0]
  BCM_ON -> EPO [order 3] : after(2,sec)[T_30C==0||CriticalBattError||MO_Fehler_Notentladung_Anf]
  data: on_plug input boolean; timer local double; tloop parameter double; T_15 input double; T_30 input double; MO_BMS_Sollmodus input double; T_30C input double; BMS_Init_abgeschlossen output double; BMS_IstModus output double; BMS_Fehler_Pilot output double; NMH_Normal_Mode_1 output double; BMS_Fehler_HS_offen output double; BMS_Fehler_HS_verschweisst output double; NMH_BMS_Start_2 output double; NMH_BMS_Start_1 output double; BMS_Fehler_Notabschaltung_Crash output double; BMS_Fehler_Notabschaltung_Pilot output double; NHM_BMS_Car_WakeUp output double; BMS_SleepInd output double; NMH_BMS_Normal_Mode_2 output double; MO_Fehler_Notentladung_Anf input double; Diag_Rq_Fktnl_Data_OBD input boolean; BattError input boolean; CriticalBattError input boolean; BMS_Fehler_HVBatt_Abschaltung output double; BMS_Fehler_HVBatt_Abschaltung_Anf output double

== stateflow chart P2_SIL_Model_Diag/Camaro Plant Model/Transmission1/Soft TCM/6L45 Logic ==
  settings: sampleTime=0.04
  state Torque_Converter_Control [parallel]
    du:
    du:[lockup_thrsh]=calc_lockup(Gear_D, drvAPP);
    du:[unlock_thrsh]=calc_unlock(Gear_D, drvAPP);
    settings: executionOrder=1
    state lockup_th = calc_lockup(Gear, APP) [function]
    note: Lever Position:
        | 1 P
        | 2 R
        | 3 N
        | 4 D
        |
        | 1 clutch lock-up
        | 0 clutch unlock
    state Lock
      en:
      LockupCmd = 1;
    state Unlock
      en:
      LockupCmd = 0;
    state unlock_th = calc_unlock(Gear,APP) [function]
    (default) -> Unlock
    Unlock -> Lock : [(Gear_D >= 4 || drvBPP > 0) && VehicleSpeed > 20]
    Lock -> Unlock : [VehicleSpeed < 20 || drvBPP == 0 && drvAPP > 5 && Gear_D <= 3]
  state Gearbox_Control [parallel]
    settings: executionOrder=2
    state Shifter_Actuator [parallel]
      settings: executionOrder=1
      state Shifter_D
        du:
        TransEstGear = Gear_D;
      state Shifter_R
        en:
        TransEstGear = 14;
      state Shifter_N
        en:
        TransEstGear = 13;
      state Shifter_P
        en:
        TransEstGear = 15;
      (default) -> Shifter_P
      Shifter_D -> Shifter_N : [ShftLvrPos <= 3]
      Shifter_N -> Shifter_R [order 2] : [ShftLvrPos <= 2]
      Shifter_R -> Shifter_P [order 2] : [ShftLvrPos <= 1]
      Shifter_N -> Shifter_D [order 1] : [ShftLvrPos >= 4]
      Shifter_R -> Shifter_N [order 1] : [ShftLvrPos >= 3]
      Shifter_P -> Shifter_R : [ShftLvrPos >= 2]
    state Shift_Schedule [parallel]
      settings: executionOrder=2
      state Gear_State_D [parallel]
        settings: executionOrder=1
        state Gear_4th
          entry:
          Gear_D = 4;
        state Gear_3rd
          entry:
          Gear_D = 3;
        state Gear_6th
          entry:
          Gear_D = 6;
        state Gear_7th
          entry:
          Gear_D = 7;
        state Gear_8th
          entry:
          Gear_D = 8;
        state Gear_1st
          entry:
          Gear_D = 1;
        state Gear_5th
          entry:
          Gear_D = 5;
        state Gear_2nd
          entry:
          Gear_D  = 2;
        (default) -> Gear_1st
        Gear_2nd -> Gear_3rd [order 1] : UP
        Gear_7th -> Gear_8th [order 1] : UP
        Gear_4th -> Gear_5th [order 1] : UP
        Gear_5th -> Gear_6th [order 1] : UP
        Gear_6th -> Gear_7th [order 1] : UP
        Gear_3rd -> Gear_4th [order 1] : UP
        Gear_1st -> Gear_2nd : UP
        Gear_3rd -> Gear_2nd [order 2] : DOWN
        Gear_4th -> Gear_3rd [order 2] : DOWN
        Gear_2nd -> Gear_1st [order 2] : DOWN
        Gear_5th -> Gear_4th [order 2] : DOWN
        Gear_6th -> Gear_5th [order 2] : DOWN
        Gear_7th -> Gear_6th [order 2] : DOWN
        Gear_8th -> Gear_7th : DOWN
      state Gear_Transient_D [parallel]
        du:[up_thrsh]=calc_up(Gear_D, drvAPP);
        du:[down_thrsh]=calc_down(Gear_D, drvAPP);
        settings: executionOrder=2
        state steady_state
        state upshifting
        state downshifting
        (default) -> steady_state
        steady_state -> upshifting [order 1] : [VehicleSpeed > up_thrsh && Gear_D < 6]
        steady_state -> downshifting [order 2] : [VehicleSpeed < down_thrsh && Gear_D > 1]
        downshifting -> steady_state [order 2] : [VehicleSpeed > down_thrsh]
        downshifting -> steady_state [order 1] : after(0.1,sec)
            | [VehicleSpeed <= down_thrsh]
            | {Gear_State_D.DOWN;}
        upshifting -> steady_state [order 1] : after(0.1,sec)
            | [VehicleSpeed >= up_thrsh]
            | {Gear_State_D.UP;}
        upshifting -> steady_state [order 2] : [VehicleSpeed < up_thrsh]
      state PlotShiftSchedule [function]
      state up_th = calc_up(Gear, APP) [function]
      state down_th = calc_down(Gear, APP) [function]
  data: Gear function_input; APP function_input; lockup_th function_output; Gear function_input; APP function_input; unlock_th function_output; Gear function_input; APP function_input; up_th function_output; Gear function_input; APP function_input; down_th function_output; tc_lockup_thrsh input double; Gear_D local int8 =1; drvAPP input double [0..100]; VehicleSpeed input double; TransEstGear output int8; down_thrsh local double =0; up_thrsh local double =0; LockupCmd output boolean; tc_spd_in input double; tc_spd_out input double; drvBPP input double; ShftLvrPos input int8; lockup_thrsh local double; unlock_thrsh local double
  events: DOWN local EITHER_EDGE_EVENT; UP local EITHER_EDGE_EVENT

== stateflow chart P2_SIL_Model_Diag/Camaro Plant Model/ICE Simple1/Engine Plant Modified/Core Engine/Crank Process ==
  state Starter_Crank
    du:
    EngActTrq = function(EngSpd_RPM);
  state Eng_Off
    du:
    EngActTrq = 0;
  state Eng_Combustion
    du:
    EngActTrq = 100;
  state CrankTrq = function(EngSpd) [function]
  state Eng_Run
    du:
    EngActTrq = EngBrkTrq;
  (default) -> Eng_Off
  Eng_Off -> Starter_Crank : [EngCrankCmd]
  Starter_Crank -> Eng_Off [order 2] : [!EngCrankCmd]
  Eng_Run -> Eng_Off : [AvlblFuel <= 0.01|| EngShutdown == 1]
  Starter_Crank -> Eng_Combustion [order 1] : after(0.5,sec)
      | [AvlblFuel >= 0.1]
  Eng_Combustion -> Eng_Run : [EngRunAtv]
  data: CrankTrq function_output; EngSpd function_input; EngRunAtv input boolean; AvlblFuel input double; EngActTrq output double; EngCrankCmd input boolean; EngBrkTrq input double; EngSpd_RPM input double; EngShutdown input boolean

== stateflow chart P2_SIL_Model_Diag/Camaro Plant Model/ICE Simple1/Soft ECM/Logic ==
  state Eng_Crank
    en:
    EngCrankCmd = 1;
    FuelPumpEnable = 1;
    EngShutdown = 0;
  state Eng_Off
    en:
    EngRunAtv = 0;
    EngCrankCmd = 0
    ThrottleCmd = 0;
    FuelPumpEnable = 0;
  state Eng_On
    en:
    EngRunAtv = 1;
    EngCrankCmd = 0;
    du:
    ThrottleCmd = APP2TP(EngSpd_RPM,drvAPP,ShftLvrPos);
  state TP = APP2TP(EngSpd,APP,Shifter) [function]
  (default) -> Eng_Off
  Eng_Off -> Eng_Crank : [SysPwrMd == 3]
  Eng_Crank -> Eng_Off [order 2] : [SysPwrMd < 3]
  Eng_On -> Eng_Off : [SysPwrMd < 2 || EngSpd_RPM < 500]
      | {EngShutdown = 1; }
  Eng_Crank -> Eng_On [order 1] : [EngSpd_RPM >= 580]
  data: EngSpd function_input; TP function_output; APP function_input; Shifter function_input; drvAPP input; ThrottleCmd output double; EngCrankCmd output boolean; SysPwrMd input int8; ShftLvrPos input int8; EngSpd_RPM input double; VehSpdAvgDrvn input double; EngRunAtv output boolean; FuelPumpEnable output double; EngShutdown output boolean

== stateflow chart P2_SIL_Model_Diag/Controller/HSC/Powertrain Manager/HV Manager/BMS_Manager/ESS_Manager ==
  state EPO
    state Open_Contactors_EPO
      entry: MO_BMS_Sollmodus=0;
      HV_State=-7;
    (default) -> Open_Contactors_EPO
  state HV_Startup
    state Drive_State
      entry:  HV_State=1;
      veh_wake=0;
      T_15=0;
      T_30=0;
      HVDischarge=0;
      timer=0;
      timer = timer + 1;
      HV_State=1;
    state Clear_Faults
      entry:
      Diag_Rq_Fktnl_Data_OBD_byte_0 =1;
      Diag_Rq_Fktnl_Data_OBD_byte_1=4;
      Diag_Rq_Fktnl_Data_OBD_byte_2=0;
      Diag_Rq_Fktnl_Data_OBD_byte_3=0;
      Diag_Rq_Fktnl_Data_OBD_byte_4=0;
      Diag_Rq_Fktnl_Data_OBD_byte_5=0;
      Diag_Rq_Fktnl_Data_OBD_byte_6=0;
      Diag_Rq_Fktnl_Data_OBD_byte_7=0;
      HV_State=2;
    state Charge_Wake
      entry: chga_wake=1;
      HV_State=3;
    state Drive_Wake
      entry: veh_wake=1;
      HV_State=8;
    state BMS_Enable_Charge
      entry: MO_BMS_Sollmodus=0;
      T_15=1;
      T_30=1;
      HV_State=4;
    state BMS_Enable_Drive
      entry: MO_BMS_Sollmodus=0;
      T_15=1;
      T_30=1;
      HV_State=9;
    state Power_Contactors_Charge
      en: MO_BMS_Sollmodus=0;
      T_30C=1;
      HV_State=5;
    state Power_Contactors_Drive
      en: MO_BMS_Sollmodus=0;
      T_30C=1;
      HV_State=10;
    state Close_Contactors_Charge
      entry:
      MO_BMS_Sollmodus=4;
      HV_State=6;
    state Close_Contactors_Drive
      entry:
      MO_BMS_Sollmodus=1;
      HV_State=11;
    state Ready_to_Charge
      entry: ReadyToCharge=1;
      HV_State=7;
    state Ready_to_Drive
      entry: ReadyToDrive=1;
      HV_State=12;
    (default) -> Drive_State
    Drive_State -> Clear_Faults
    Clear_Faults -> Charge_Wake [order 1] : [plugged]
    Clear_Faults -> Drive_Wake [order 2] : after(0.1,sec)
    Drive_Wake -> BMS_Enable_Drive : after(0.1,sec)[BMS_Fehler_Pilot==0 ]
    Charge_Wake -> BMS_Enable_Charge : [BMS_Fehler_Pilot==0 ]
    BMS_Enable_Charge -> Power_Contactors_Charge : [BMS_Init_abgeschlossen]
    BMS_Enable_Drive -> Power_Contactors_Drive : after(0.1,sec)[BMS_Init_abgeschlossen]
    Power_Contactors_Charge -> Close_Contactors_Charge : [closeMaincReq]
    Power_Contactors_Drive -> Close_Contactors_Drive : [closeMaincReq]
    Close_Contactors_Charge -> Ready_to_Charge : [BMS_Fehler_HS_offen==0&&BMS_IstModus==3]
    Close_Contactors_Drive -> Ready_to_Drive : [BMS_Fehler_HS_offen==0&&BMS_IstModus==1]
  state HV_Shudown
    state Open_Contactors
      entry: MO_BMS_Sollmodus=0;
      T_30C=0;
      HV_State=-1;
    state Discharge_Bus
      entry: HVDischarge=1;
      HV_State=-2;
    state Disable_BCM_1
      entry: T_15=0;
      HVDischarge=0;
      HV_State=-3;
    state Disable_BCM_2
      entry: T_30=0;
      HVDischarge=0;
      HV_State=-4;
    state Send_BCM_to_Sleep
      en: MO_SleepAckn =1;
      T_15=0;
      T_30=0;
      T_30C=0;
      HV_State=-5;
    state Shutdown_Complete
      entry: Shutdown_Complete=1;
      HV_State=-6;
    (default) -> Open_Contactors : [~closeMaincReq]
    Open_Contactors -> Discharge_Bus : [BMS_IstModus==5]
    Discharge_Bus -> Disable_BCM_1 : [BMS_Spannung_ZwKr<30]
    Disable_BCM_1 -> Disable_BCM_2 : [BMS_IstStrom<0.02]
    Disable_BCM_2 -> Send_BCM_to_Sleep
    Send_BCM_to_Sleep -> Shutdown_Complete : [BMS_SleepInd]
  note: NEEDS REVISION
  note: Need to add a state into Shutdown to wait for all the HV components to be off
      | before opening contactors
  note: Need  to check what's the IstModus value after we open contactors to put it
      | as transition between open contactors and discharge bus
  note: 
  HV_Startup -> EPO [order 2] : [ISOfault==1]
  EPO -> HV_Shudown : [ISOfault==0]
  (default) -> HV_Shudown
  HV_Shudown -> HV_Startup : [HV_req==1]
  HV_Startup -> HV_Shudown [order 1] : [HV_req==0]
      | {ReadyToCharge=0;
      | ReadyToDrive=0;}
  data: data local; ISOfault input; plugged input; BMS_Fehler_HS_offen input; BMS_Fehler_Pilot input; BMS_Init_abgeschlossen input; BMS_IstModus input; BMS_IstSpannung input; BMS_IstStrom input; BMS_SleepInd input; Diag_Rq_Fktnl_Data_OBD_byte_0 output; Diag_Rq_Fktnl_Data_OBD_byte_1 output; Diag_Rq_Fktnl_Data_OBD_byte_2 output; Diag_Rq_Fktnl_Data_OBD_byte_3 output; Diag_Rq_Fktnl_Data_OBD_byte_4 output; Diag_Rq_Fktnl_Data_OBD_byte_5 output; Diag_Rq_Fktnl_Data_OBD_byte_6 output; Diag_Rq_Fktnl_Data_OBD_byte_7 output; MO_SleepAckn output; MO_BMS_Sollmodus output; T_15 output; T_30 output; T_30C output; veh_wake output; chga_wake output; HVDischarge output; HV_State output; ReadyToDrive output; ReadyToCharge output; Shutdown_Complete output; HV_req input; BMS_Spannung_ZwKr input; NMH_BMS_Car_WakeUp input; NMH_Normal_Mode_1 input; NMH_BMS_Normal_Mode_2 input; NMH_BMS_Start_1 input; NMH_BMS_Start_2 input; timer local; closeMaincReq input; SysPwrMd input

== stateflow chart P2_SIL_Model_Diag/Camaro Plant Model/ICE Simple1/Soft ECM/ECM_RollingAliveCnt/Rolling Alive Counter ==
  state RollingAliveCounter
    state Count1
      en: RollingAliveCnt = 0;
    state Count2
      en: RollingAliveCnt = 1;
    state Count3
      en: RollingAliveCnt = 2;
    state Count4
      en: RollingAliveCnt = 3;
    (default) -> Count1
    Count4 -> Count1 : after(0.01,sec)
    Count1 -> Count2 : after(0.01,sec)
    Count2 -> Count3 : after(0.01,sec)
    Count3 -> Count4 : after(0.01,sec)
  data: RollingAliveCnt output int8 =0
